simulink model "practica3_simulink"  (R2023b)
settings: Solver=ode45  StartTime=0.0  StopTime=10  RelTol=1e-3
values from neighbouring files (symbols this model uses):
  b1 = 1000    [PRACTICA3.m]    (also in PRACTICA3_matlab.m; variables para simulink.mat)
  k1 = 16182    [PRACTICA3.m]    (also in PRACTICA3_matlab.m; variables para simulink.mat)
  k2 = 19000    [PRACTICA3.m]    (also in PRACTICA3_matlab.m; variables para simulink.mat)
  m1 = 290    [PRACTICA3.m]    (also in PRACTICA3_matlab.m; variables para simulink.mat)
  m2 = 59    [PRACTICA3.m]    (also in PRACTICA3_matlab.m; variables para simulink.mat)
settings Model: Creator=lombo  LastModifiedBy=lombo

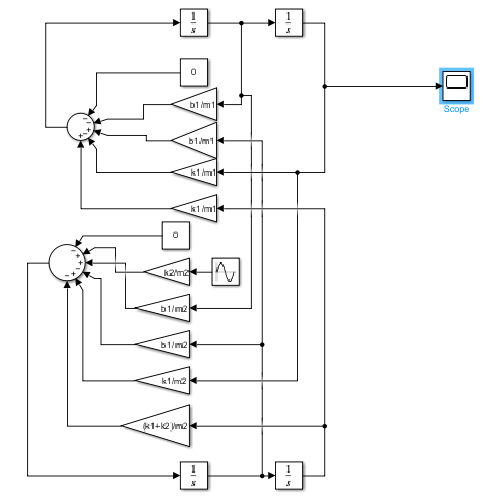
[thumbnail: Simulink's stored preview of the top-level diagram]
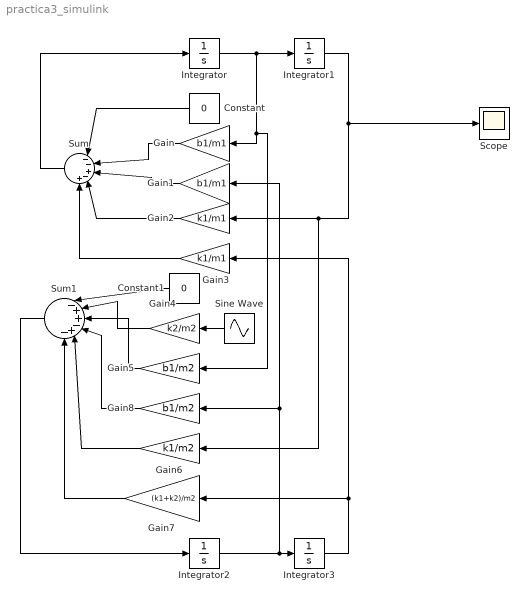
== system practica3_simulink ==
  Constant : Constant  Value=0
  Constant1 : Constant  Value=0
  Gain : Gain  Gain=b1/m1
  Gain1 : Gain  Gain=b1/m1
  Gain2 : Gain  Gain=k1/m1
  Gain3 : Gain  Gain=k1/m1
  Gain4 : Gain  Gain=k2/m2
  Gain5 : Gain  Gain=b1/m2
  Gain6 : Gain  Gain=k1/m2
  Gain7 : Gain  Gain=(k1+k2)/m2
  Gain8 : Gain  Gain=b1/m2
  Integrator{,1..3} (4 alike) : Integrator
  Scope : Scope
  Sine Wave : Sin  Amplitude=0.05  Frequency=0.5*pi  SampleTime=0
  Sum : Sum  Inputs=|--+-+
  Sum1 : Sum  Inputs=|-++-+-
  wires:
  Integrator/1 -> Gain5/1, Gain/1, Integrator1/1
  Integrator2/1 -> Gain8/1, Gain1/1, Integrator3/1
  Integrator1/1 -> Gain6/1, Gain2/1, Scope/1
  Integrator3/1 -> Gain3/1, Gain7/1
  Constant/1 -> Sum/1
  Gain/1 -> Sum/2
  Gain1/1 -> Sum/3
  Gain2/1 -> Sum/4
  Gain3/1 -> Sum/5
  Sum/1 -> Integrator/1
  Sine Wave/1 -> Gain4/1
  Constant1/1 -> Sum1/1
  Sum1/1 -> Integrator2/1
  Gain4/1 -> Sum1/2
  Gain5/1 -> Sum1/3
  Gain8/1 -> Sum1/4
  Gain6/1 -> Sum1/5
  Gain7/1 -> Sum1/6
